simulink model "modelo_simulink_ros"  (R2019b)
settings: Solver=FixedStepDiscrete  StartTime=0.0  StopTime=100.0  FixedStep=0.1  RelTol=1e-3
undefined symbols (not defined in the file or in its folder): Angular, Linear
libraries: robotlib x3, dspsigops x2, simulink x1
settings Model: SimulationMode=external  Creator=Pablo  LastModifiedBy=Pablo
settings OptimizationCC: EnhancedBackFolding=on  PassReuseOutputArgsAs=Individual arguments  ZeroExternalMemoryAtStartup=off  ZeroInternalMemoryAtStartup=off  MaxStackSize=64  OptimizeBlockOrder=speed  DifferentSizesBufferReuse=on  OptimizationCustomize=off  EfficientTunableParamExpr=on
settings DebuggingCC: ParameterTunabilityLossMsg=error
settings HardwareCC: ProdBitPerPointer=32  ProdBitPerSizeT=32  ProdBitPerPtrDiffT=32  ProdLargestAtomicFloat=None  ProdIntDivRoundTo=Undefined  ProdEndianess=Unspecified  ProdWordSize=32  ProdHWDeviceType=Generic->Unspecified (assume 32-bit Generic)  UseEmbeddedCoderFeatures=off
settings SFSimCC: MATLABDynamicMemAlloc=off
settings RTWCC: SystemTargetFile=ert.tlc  HardwareBoard=Robot Operating System (ROS)  TLCOptions="-aInlineSetEventsForThisBaseRateFcn=TLC_FALSE -aSuppressMultiTaskScheduler=TLC_FALSE  -aRateBasedStepFcn=0"  TemplateMakefile=ert_default_tmf  GenerateReport=on  Toolchain=Catkin  IncludeHyperlinkInReport=on  LaunchReport=on  TargetLang=C++  GenerateTraceInfo=on  GenerateTraceReport=on  GenerateTraceReportSl=on  GenerateTraceReportSf=on  GenerateTraceReportEml=on
settings CodeAppCC: ForceParamTrailComments=on  IgnoreCustomStorageClasses=off  OperatorAnnotations=on  SimulinkDataObjDesc=on  SFDataObjDesc=on  InsertBlockDesc=on
settings ERTTargetCC: SupportNonInlinedSFcns=on

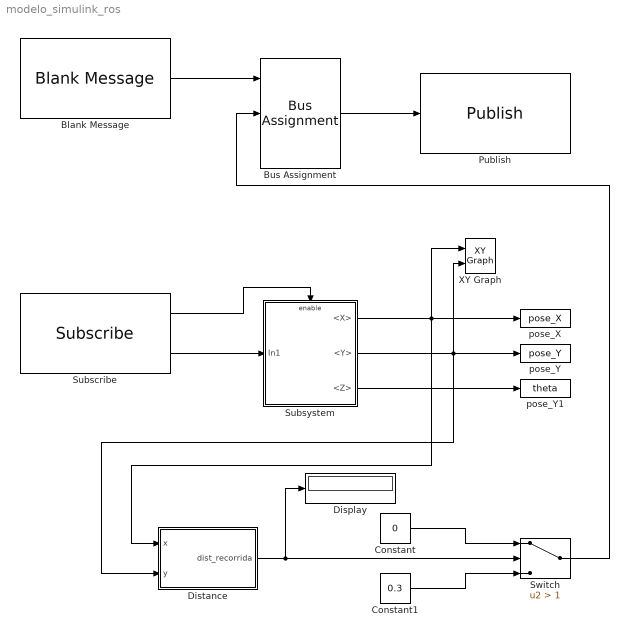
== system modelo_simulink_ros ==
  Blank Message : robotlib/Blank Message  messageClass=Message  entityType=geometry_msgs/Twist  messageType=geometry_msgs/Twist  SampleTime=inf
      settings: SourceProductName=ROS Toolbox
  Bus Assignment : BusAssignment  AssignedSignals=Linear.X,Angular.Z
  Constant : Constant  Value=0
  Constant1 : Constant  Value=0.3
  Display : Display
  Distance : Subsystem
  Publish : robotlib/Publish  topicSource=Select from ROS network  topic=/robot0/cmd_vel  messageType=geometry_msgs/Twist  messageQueueLength=1
      settings: SourceProductName=ROS Toolbox
  Subscribe : robotlib/Subscribe  topicSource=Select from ROS network  topic=/robot0/odom  messageType=nav_msgs/Odometry  sampleTime=-1  messageQueueLength=1
      settings: SourceProductName=ROS Toolbox
  Subsystem : Subsystem
  Switch : Switch  Criteria=u2 > Threshold  Threshold=1
  XY Graph : simulink/Sinks/XY Graph  xmin=-100  xmax=100  ymin=-100  ymax=100  st=-1
  pose_X : ToWorkspace  VariableName=pose_X  SampleTime=-1
      settings: Save2DSignal=2-D array (concatenate along first dimension)
  pose_Y : ToWorkspace  VariableName=pose_Y  SampleTime=-1
      settings: Save2DSignal=2-D array (concatenate along first dimension)
  pose_Y1 : ToWorkspace  VariableName=theta  SampleTime=-1
      settings: Save2DSignal=2-D array (concatenate along first dimension)
  wires:
  Blank Message/1 -> Bus Assignment/1
  Bus Assignment/1 -> Publish/1
  Subscribe/2 -> Subsystem/1(In1)
  Subscribe/1 -> Subsystem/Enable
  Subsystem/1(<X>) -> Distance/1(x), XY Graph/1, pose_X/1
  Subsystem/2(<Y>) -> Distance/2(y), XY Graph/2, pose_Y/1
  Subsystem/3(<Z>) -> pose_Y1/1
  Distance/1(dist_recorrida) -> Display/1, Switch/2
  Switch/1 -> Bus Assignment/2
  Constant1/1 -> Switch/3
  Constant/1 -> Switch/1

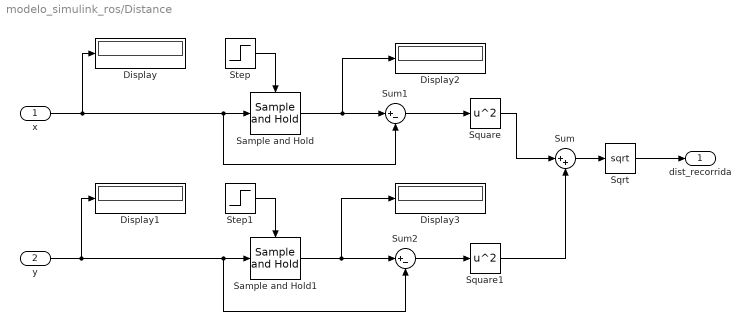
== system modelo_simulink_ros/Distance ==
  x : Inport
  y : Inport  Port=2
  Display{,1..3} (4 alike) : Display
  Sample and Hold : dspsigops/Sample and Hold  trig=Rising edge  initCond=0  latchinput=off
  Sample and Hold1 : dspsigops/Sample and Hold  trig=Rising edge  initCond=0  latchinput=off
  Sqrt : Sqrt  SaturateOnIntegerOverflow=on
  Square : Math  Operator=square  SignedPower=off  SaturateOnIntegerOverflow=on
  Square1 : Math  Operator=square  SignedPower=off  SaturateOnIntegerOverflow=on
  Step : Step  SampleTime=0
  Step1 : Step  SampleTime=0
  Sum : Sum  Inputs=|++
  Sum1 : Sum  Inputs=|+-
  Sum2 : Sum  Inputs=|+-
  dist_recorrida : Outport
  wires:
  Sum2/1 -> Square1/1
  Step/1 -> Sample and Hold/Trigger
  Sample and Hold/1 -> Display2/1, Sum1/1
  Sqrt/1 -> dist_recorrida/1
  Square1/1 -> Sum/2
  x/1 -> Display/1, Sum1/2, Sample and Hold/1
  Square/1 -> Sum/1
  y/1 -> Display1/1, Sum2/2, Sample and Hold1/1
  Sum/1 -> Sqrt/1
  Sample and Hold1/1 -> Display3/1, Sum2/1
  Sum1/1 -> Square/1
  Step1/1 -> Sample and Hold1/Trigger

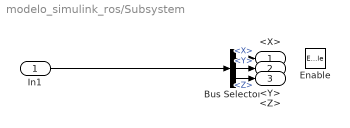
== system modelo_simulink_ros/Subsystem ==
  In1 : Inport
  Enable : EnablePort
  Bus Selector : BusSelector  OutputSignals=Pose.Pose.Position.X,Pose.Pose.Position.Y,Pose.Pose.Orientation.Z
  <X> : Outport
  <Y> : Outport  Port=2
  <Z> : Outport  Port=3
  wires:
  Bus Selector/1 -> <X>/1  "<X>"
  Bus Selector/2 -> <Y>/1  "<Y>"
  Bus Selector/3 -> <Z>/1  "<Z>"
  In1/1 -> Bus Selector/1
